simulink model "microgrid"  (R2023b)
settings: Solver=VariableStepAuto  StartTime=0.0  StopTime=120  FixedStep=1e-5  MaxStep=0.0055555555555555558  RelTol=1e-3
undefined symbols (not defined in the file or in its folder): D11, Delta
libraries: spsThreePhaseVIMeasurementLib x3, spsDistributedParametersLineLib x2, spsGroundLib x2, spsThreePhaseTransformerTwoWindingsLib x2, spsThreePhaseSourceLib x2, spsMultimeterLib x1, spsThreePhaseSeriesRLCLoadLib x1, spsThreePhaseFaultLib x1, spspowerguiLib x1
settings Model: Creator=62614  LastModifiedBy=62614
settings DataIOCC: SaveFinalState=on  SaveState=on  LoggingToFile=on
settings HardwareCC: TargetBitPerPointer=64  TargetBitPerSizeT=64  TargetBitPerPtrDiffT=64  TargetLargestAtomicFloat=Float  TargetIntDivRoundTo=Zero  TargetEndianess=LittleEndian  TargetWordSize=64  TargetHWDeviceType=Intel->x86-64 (Windows64)  ProdEqTarget=off

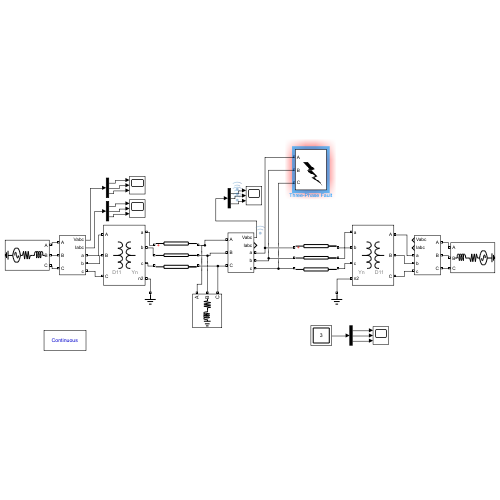
[thumbnail: Simulink's stored preview of the top-level diagram]
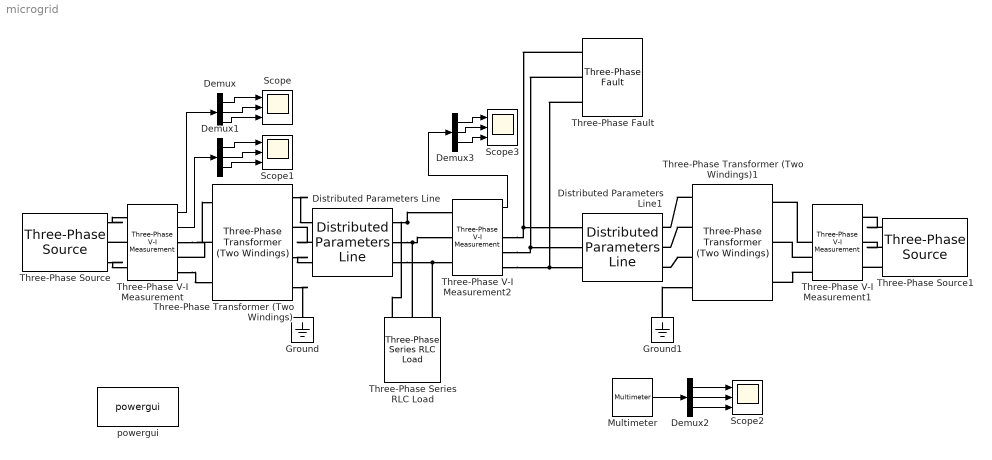
== system microgrid ==
  Demux{,1..3} (4 alike) : Demux  Outputs=3
  Distributed Parameters Line : spsDistributedParametersLineLib/Distributed Parameters Line  Phases=3  Length=20  Frequency=60  Resistance=[0.01273 0.3864]  Inductance="[0.9337e-3  4.1264e-3]"  Capacitance=[12.74e-9 7.751e-9]  x1=[1.028975793723e-11 112687.987262361 112687.987262358;376.991118430775 376.991118430775 376.991118430775;-0.828038992969612 -0.0490320013081402 -1.61982832810305]  x2=[2.99244834855497e-11 112733.855552849 112733.855552847;376.991118430775 376.991118430775 376.991118430775;2.59111531237921 -0.0490794534441862 -1.6198757802391]  x3=[1.11271701725279e-12 415.608924474705 415.608924474687;376.991118430775 376.991118430775 376.991118430775;1.79162203825765 -0.077769790234125 -1.64856611702906]  x4=[3.57213295306242e-12 416.654634078014 416.654634078009;376.991118430775 376.991118430775 376.991118430775;-2.90355570735577 -0.0463917770390216 -1.6171881038339]  x5=0.000113108313399148  V1=[1.029e-11 1.127e+05 1.127e+05;377 377 377;-0.828 -0.04903 -1.62]  V2=[2.992e-11 1.127e+05 1.127e+05;377 377 377;2.591 -0.04908 -1.62]  I1=[1.113e-12 415.6 415.6;377 377 377;1.792 -0.07777 -1.649]  I2=[3.572e-12 416.7 416.7;377 377 377;-2.904 -0.04639 -1.617]  nHarmo=1  Measurements=None  Decoupling=off  VsMag0=0  VrMag0=0  VsAngle0=0  VrAngle0=0  IsMag0=0  IrMag0=0  IsAngle0=0  IrAngle0=0
      settings: LibrarySourceBlock=sps_lib/Power Grid Elements/Distributed Parameters Line
  Distributed Parameters Line1 : spsDistributedParametersLineLib/Distributed Parameters Line  Phases=3  Length=25  Frequency=60  Resistance=[0.01273 0.3864]  Inductance="[0.9337e-3  4.1264e-3]"  Capacitance=[12.74e-9 7.751e-9]  x1=[3.25390716534427e-11 112733.855552849 112733.855552847;376.991118430775 376.991118430775 376.991118430775;2.62464400762378 -0.0555805934134384 -1.62637692020835]  x2=[1.40971678774804e-11 112688.424260216 112688.424260213;376.991118430775 376.991118430775 376.991118430775;3.08829161662459 -0.0555252750884904 -1.6263216018834]  x3=[1.36200714849201e-12 416.58049063166 416.58049063165;376.991118430775 376.991118430775 376.991118430775;2.85823956324716 -0.0593860340164718 -1.6301823608114]  x4=[1.30815763671597e-12 415.539491563043 415.539491563029;376.991118430775 376.991118430775 376.991118430775;1.95338901321701 -0.0842662267583654 -1.65506255355327]  x5=0.000141385391748936  V1=[3.254e-11 1.127e+05 1.127e+05;377 377 377;2.625 -0.05558 -1.626]  V2=[1.41e-11 1.127e+05 1.127e+05;377 377 377;3.088 -0.05553 -1.626]  I1=[1.362e-12 416.6 416.6;377 377 377;2.858 -0.05939 -1.63]  I2=[1.308e-12 415.5 415.5;377 377 377;1.953 -0.08427 -1.655]  nHarmo=1  Measurements=None  Decoupling=off  VsMag0=0  VrMag0=0  VsAngle0=0  VrAngle0=0  IsMag0=0  IrMag0=0  IsAngle0=0  IrAngle0=0
      settings: LibrarySourceBlock=sps_lib/Power Grid Elements/Distributed Parameters Line
  Ground : spsGroundLib/Ground  LConnTagsString=a
  Ground1 : spsGroundLib/Ground  LConnTagsString=a
  Multimeter : spsMultimeterLib/Multimeter  L=6  sel=[1 2 3]  yselected={}  Gain=[1 1 1]  OutputType=Complex  PlotAtSimulationStop=off  PhasorSimulation=off
  Scope{,1..3} (4 alike) : Scope  NumInputPorts=3
  Three-Phase Series RLC Load : spsThreePhaseSeriesRLCLoadLib/Three-Phase Series RLC Load  LConnTagsString=A|B|C  Configuration=Y (grounded)  NominalVoltage=110e3  Vabc=[1e3 1e3 1e3]  Vabcp=[1e3 1e3 1e3]  NominalFrequency=60  UnbalancedPower=off  ActivePower=100e3  InductivePower=50e3  CapacitivePower=0  Pabc=[10e3 9e3 11e3]  QLabc=[100 90 110]  QCabc=[100 90 110]  Pabcp=[10e3 9e3 11e3]  QLabcp=[100 90 110]  QCabcp=[100 90 110]  Measurements=None  LoadType=constant Z
  Three-Phase Transformer (Two Windings) : spsThreePhaseTransformerTwoWindingsLib/Three-Phase Transformer (Two Windings)  Winding1Connection=Delta (D11)  Winding2Connection=Yn  CoreType=Three single-phase transformers  SetSaturation=off  Hysteresis=off  DataFile='hysteresis'  SetInitialFlux=off  Measurements=None  UNITS=pu  NominalPower=[ 250e6 , 60 ]  Winding1=[ 10.5e3 , 0.002 , 0.08 ]  Winding2=[ 110e3 , 0.002 , 0.08 ]  Rm=500  Lm=500  L0=0.5  Saturation=[ 0,0 ; 0.0024,1.2 ; 1.0,1.52 ]  InitialFluxes=[ 0.8 , -0.8 , 0.7 ]  BreakLoop=off  DiscreteSolver=Trapezoidal iterative  DataType=off  TransfoNumber=1
  Three-Phase Transformer (Two Windings)1 : spsThreePhaseTransformerTwoWindingsLib/Three-Phase Transformer (Two Windings)  Winding1Connection=Delta (D11)  Winding2Connection=Yn  CoreType=Three single-phase transformers  SetSaturation=off  Hysteresis=off  DataFile='hysteresis'  SetInitialFlux=off  Measurements=None  UNITS=pu  NominalPower=[ 250e6 , 60 ]  Winding1=[ 10.5e3 , 0.002 , 0.08 ]  Winding2=[ 110e3 , 0.002 , 0.08 ]  Rm=500  Lm=500  L0=0.5  Saturation=[ 0,0 ; 0.0024,1.2 ; 1.0,1.52 ]  InitialFluxes=[0.8 -0.8 0.7]  BreakLoop=off  DiscreteSolver=Trapezoidal iterative  DataType=off  TransfoNumber=1
  Three-Phase V-I Measurement : spsThreePhaseVIMeasurementLib/Three-Phase V-I Measurement  VoltageMeasurement=phase-to-ground  SetLabelV=off  LabelV=Vabc  Vpu=off  VpuLL=off  CurrentMeasurement=yes  SetLabelI=off  LabelI=Iabc  Ipu=off  Pbase=100e6  Vbase=500e3  OutputType=Complex  PhasorSimulation=off  PSBequivalent=0
  Three-Phase V-I Measurement1 : spsThreePhaseVIMeasurementLib/Three-Phase V-I Measurement  VoltageMeasurement=phase-to-ground  SetLabelV=off  LabelV=Vabc  Vpu=off  VpuLL=off  CurrentMeasurement=yes  SetLabelI=off  LabelI=Iabc  Ipu=off  Pbase=100e6  Vbase=500e3  OutputType=Complex  PhasorSimulation=off  PSBequivalent=0
  Three-Phase V-I Measurement2 : spsThreePhaseVIMeasurementLib/Three-Phase V-I Measurement  VoltageMeasurement=phase-to-ground  SetLabelV=off  LabelV=Vabc  Vpu=on  VpuLL=off  CurrentMeasurement=yes  SetLabelI=off  LabelI=Iabc  Ipu=off  Pbase=100e6  Vbase=115e3  OutputType=Complex  PhasorSimulation=off  PSBequivalent=0
  Three-Phase Fault : spsThreePhaseFaultLib/Three-Phase Fault  InitialStates=0  FaultA=off  FaultB=on  FaultC=on  GroundFault=off  SwitchTimes=fault_set  External=off  SwitchStatus=NaN  FaultResistance=0.001  GroundResistance=0.01  SnubberResistance=1e6  SnubberCapacitance=inf  Measurements=Fault voltages and currents
  Three-Phase Source : spsThreePhaseSourceLib/Three-Phase Source  InternalConnection=Yg  VoltagePhases=off  Voltage=10.5e3  PhaseAngle=0  Voltage_phases=[25e3 25e3 25e3]/sqrt(3)  PhaseAngles_phases=[0 -120 +120]  Frequency=60  NonIdealSource=on  SpecifyImpedance=on  Resistance=0.8929  Inductance=16.58e-3  ShortCircuitLevel=30e6  BaseVoltage=10.5e3  XRratio=7  BusType=swing  Pref=10e3  Qref=0  Prefabc=[10e3, 10e3, 10e3]  Qrefabc=[0, 0, 0]  Qmin=-inf  Qmax=inf
  Three-Phase Source1 : spsThreePhaseSourceLib/Three-Phase Source  InternalConnection=Yg  VoltagePhases=off  Voltage=10.5e3  PhaseAngle=0  Voltage_phases=[25e3 25e3 25e3]/sqrt(3)  PhaseAngles_phases=[0 -120 +120]  Frequency=60  NonIdealSource=on  SpecifyImpedance=on  Resistance=0.8929  Inductance=16.58e-3  ShortCircuitLevel=30e6  BaseVoltage=10.5e3  XRratio=7  BusType=swing  Pref=10e3  Qref=0  Prefabc=[10e3, 10e3, 10e3]  Qrefabc=[0, 0, 0]  Qmin=-inf  Qmax=inf
  powergui : spspowerguiLib/powergui  Priority=1  SimulationMode=Continuous  SampleTime=50e-6  frequency=60  Iterations=50  frequencyindice=60  Pbase=100e6  ErrMax=1e-4  UnitsV=kV  UnitsW=MW  buscounter=0  FunctionMessages=off  echomessages=off  EnableUseOfTLC=off  CurrentSourceSwitches=off  DisableSnubberDevices=off  DisableRonSwitches=off  DisableVfSwitches=off  DisplayEquations=off  AutomaticDiscreteSolvers=off  SolverType=Tustin/Backward Euler (TBE)  Interpol=off  ExternalGateDelay=off  methode=off  Ts=100  x0status=blocks  SPID=on  SwTol=0  HookPort=off  NonlinearTolerance=1e-4  nMaxIteration=100  ContinueOnMaxIteration=off  RestoreLinks=warning  ResistiveCurrentMeasurement=off  Frange=[0:2:500]  Ylog=off  Xlog=on  ShowGrid=off  save=off  variable=ZData  structure=0  ZoomFFT=off  StartTime=0.0  cycles=1  DisplayStyle=1  fundamental=60  FreqAxis=off  MaxFrequency=1000  frequencyindicesteady=1  RmsSteady=1  display=off
  wires:
  Three-Phase V-I Measurement/1 -> Demux/1
  Demux/1 -> Scope/1
  Demux/2 -> Scope/2
  Demux/3 -> Scope/3
  Demux1/1 -> Scope1/1
  Demux1/2 -> Scope1/2
  Demux1/3 -> Scope1/3
  Three-Phase V-I Measurement/2 -> Demux1/1
  Multimeter/1 -> Demux2/1
  Demux2/1 -> Scope2/1
  Demux2/2 -> Scope2/2
  Demux2/3 -> Scope2/3
  Demux3/1 -> Scope3/1
  Demux3/2 -> Scope3/2
  Demux3/3 -> Scope3/3
  Three-Phase V-I Measurement2/1 -> Demux3/1
  connections:
  Distributed Parameters Line/LConn2 -- Three-Phase Transformer (Two Windings)/RConn2
  Three-Phase V-I Measurement/LConn2 -- Three-Phase Source/RConn2
  Three-Phase Source/RConn1 -- Three-Phase V-I Measurement/LConn1
  Three-Phase Source/RConn3 -- Three-Phase V-I Measurement/LConn3
  Three-Phase V-I Measurement/RConn1 -- Three-Phase Transformer (Two Windings)/LConn1
  Three-Phase V-I Measurement/RConn3 -- Three-Phase Transformer (Two Windings)/LConn3
  Three-Phase Transformer (Two Windings)/RConn1 -- Distributed Parameters Line/LConn1
  Three-Phase Transformer (Two Windings)/RConn3 -- Distributed Parameters Line/LConn3
  Three-Phase Source1/RConn1 -- Three-Phase V-I Measurement1/LConn1
  Three-Phase Source1/RConn2 -- Three-Phase V-I Measurement1/LConn2
  Three-Phase Source1/RConn3 -- Three-Phase V-I Measurement1/LConn3
  Three-Phase Transformer (Two Windings)/RConn4 -- Ground/LConn1
  Three-Phase V-I Measurement1/RConn1 -- Three-Phase Transformer (Two Windings)1/LConn1
  Three-Phase V-I Measurement1/RConn2 -- Three-Phase Transformer (Two Windings)1/LConn2
  Three-Phase V-I Measurement1/RConn3 -- Three-Phase Transformer (Two Windings)1/LConn3
  Three-Phase Transformer (Two Windings)1/RConn1 -- Distributed Parameters Line1/RConn1
  Three-Phase Transformer (Two Windings)1/RConn2 -- Distributed Parameters Line1/RConn2
  Three-Phase Transformer (Two Windings)1/RConn3 -- Distributed Parameters Line1/RConn3
  Ground1/LConn1 -- Three-Phase Transformer (Two Windings)1/RConn4
  Three-Phase Fault/LConn1 -- Three-Phase V-I Measurement2/RConn1 -- Distributed Parameters Line1/LConn1
  Three-Phase Fault/LConn2 -- Three-Phase V-I Measurement2/RConn2 -- Distributed Parameters Line1/LConn2
  Three-Phase Fault/LConn3 -- Three-Phase V-I Measurement2/RConn3 -- Distributed Parameters Line1/LConn3
  Three-Phase Transformer (Two Windings)/LConn2 -- Three-Phase V-I Measurement/RConn2
  Distributed Parameters Line/RConn1 -- Three-Phase Series RLC Load/LConn1 -- Three-Phase V-I Measurement2/LConn1
  Distributed Parameters Line/RConn2 -- Three-Phase Series RLC Load/LConn2 -- Three-Phase V-I Measurement2/LConn2
  Distributed Parameters Line/RConn3 -- Three-Phase Series RLC Load/LConn3 -- Three-Phase V-I Measurement2/LConn3
